simulink model "kinematics_subsytem"  (R2015a)
settings: Solver=ode45  StartTime=0.0  StopTime=10.0  RelTol=1e-3
libraries: fl_lib x16
settings Model: Creator=Sourabh Khemka  LastModifiedBy=Sourabh Khemka

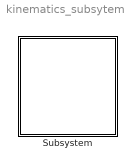
== system kinematics_subsytem ==
  Subsystem : Subsystem

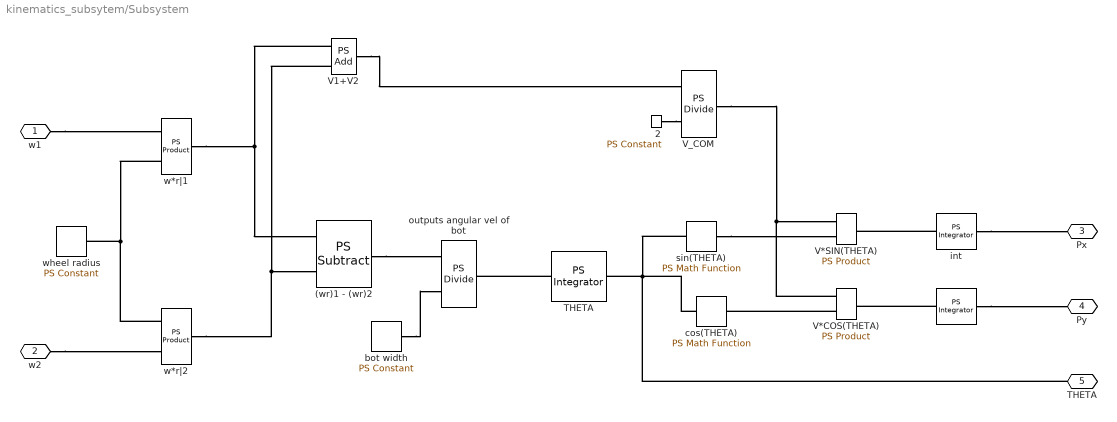
== system kinematics_subsytem/Subsystem ==
  " " : fl_lib/Physical Signals/Linear Operators/PS Integrator  x0=0
  " THETA " : fl_lib/Physical Signals/Linear Operators/PS Integrator  x0=0
  "(wr)1 - (wr)2 " : fl_lib/Physical Signals/Functions/PS Subtract
  2 : fl_lib/Physical Signals/Sources/PS Constant  constant=2
  V*COS(THETA) : fl_lib/Physical Signals/Functions/PS Product
  V*SIN(THETA) : fl_lib/Physical Signals/Functions/PS Product
  "V1+V2 " : fl_lib/Physical Signals/Functions/PS Add
  V_COM : fl_lib/Physical Signals/Functions/PS Divide
  "bot width " : fl_lib/Physical Signals/Sources/PS Constant  constant=1
  cos(THETA) : fl_lib/Physical Signals/Functions/PS Math Function  fcn_choice=2
  int : fl_lib/Physical Signals/Linear Operators/PS Integrator  x0=0
  outputs angular vel of bot : fl_lib/Physical Signals/Functions/PS Divide
  sin(THETA) : fl_lib/Physical Signals/Functions/PS Math Function  fcn_choice=1
  w*r|1 : fl_lib/Physical Signals/Functions/PS Product
  "w*r|2 " : fl_lib/Physical Signals/Functions/PS Product
  "wheel radius " : fl_lib/Physical Signals/Sources/PS Constant  constant=1
  "w1 " : PMIOPort  Port=1  Side=Left
  w2 : PMIOPort  Port=2  Side=Right
  Px : PMIOPort  Port=3  Side=Left
  Py : PMIOPort  Port=4  Side=Right
  THETA : PMIOPort  Port=5  Side=Left
  connections:
  "w1 "/RConn1 -- w*r|1/LConn1
  w*r|1/LConn2 -- "w*r|2 "/LConn1 -- "wheel radius "/RConn1
  w2/RConn1 -- "w*r|2 "/LConn2
  "V1+V2 "/RConn1 -- V_COM/LConn1
  " THETA "/LConn1 -- outputs angular vel of bot/RConn1
  " "/LConn1 -- V*COS(THETA)/RConn1
  2/RConn1 -- V_COM/LConn2
  "(wr)1 - (wr)2 "/RConn1 -- outputs angular vel of bot/LConn1
  V*COS(THETA)/LConn2 -- cos(THETA)/RConn1
  int/RConn1 -- Px/RConn1
  "bot width "/RConn1 -- outputs angular vel of bot/LConn2
  " "/RConn1 -- Py/RConn1
  sin(THETA)/RConn1 -- V*SIN(THETA)/LConn2
  "w*r|2 "/RConn1 -- "V1+V2 "/LConn2 -- "(wr)1 - (wr)2 "/LConn2
  V_COM/RConn1 -- V*COS(THETA)/LConn1 -- V*SIN(THETA)/LConn1
  w*r|1/RConn1 -- "V1+V2 "/LConn1 -- "(wr)1 - (wr)2 "/LConn1
  int/LConn1 -- V*SIN(THETA)/RConn1
  sin(THETA)/LConn1 -- THETA/RConn1 -- cos(THETA)/LConn1 -- " THETA "/RConn1
